simulink model "estimator"  (R2024b)
settings: Solver=VariableStepAuto  StartTime=0.0  StopTime=10.0  RelTol=1e-6
undefined symbols (not defined in the file): i, init, o
settings Model: Creator=jefft  LastModifiedBy=jefft
settings SFSimCC: SimCustomHeaderCode="#include \"estimator.h\""  SimTargetLang=C++
settings SFSimCC: SimUserSources=|
  | MathFunctions.cpp
  | MEKF.cpp
  | MEKFEstimatorModule.cpp
  | estimator.cpp
settings SFSimCC: SimUserIncludeDirs=|
  | ../lib/math
  | ../lib/estimator
  | ../lib/error
  | ../lib/flightmodule
settings RTWCC: GPUComputeCapability=3.5

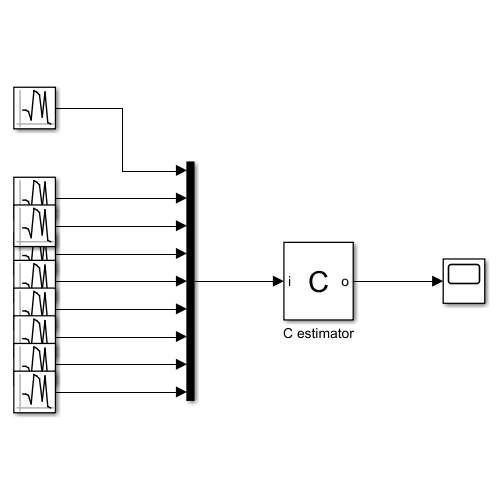
[thumbnail: Simulink's stored preview of the top-level diagram]
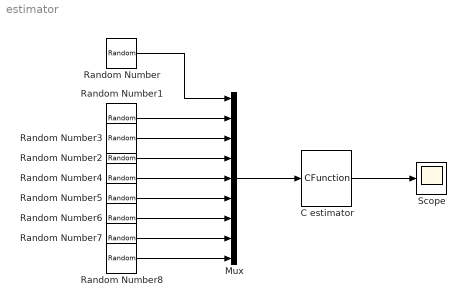
== system estimator ==
  C estimator : CFunction  OutputCode=run(i, o);  StartCode=init();  GenerateCodeAsIs=off  CodegenOutputCode=run(i, o);  CodegenStartCode=init();  CustomCodeSettingLocation=ModelConfigurationParameters
  Mux : Mux  Inputs=9
  Random Number : RandomNumber  Mean=1  Seed=1  SampleTime=0.1
  Random Number1 : RandomNumber  Mean=1  Seed=2  SampleTime=0.1
  Random Number2 : RandomNumber  Mean=1  Seed=5  SampleTime=0.1
  Random Number3 : RandomNumber  Mean=1  Seed=1  SampleTime=0.1
  Random Number4 : RandomNumber  Mean=1  SampleTime=0.1
  Random Number{5..8} (4 alike) : RandomNumber  Mean=1  Seed=6  SampleTime=0.1
  Scope : Scope
  wires:
  Mux/1 -> C estimator/1
  Random Number/1 -> Mux/1
  C estimator/1 -> Scope/1
  Random Number1/1 -> Mux/2
  Random Number2/1 -> Mux/4
  Random Number5/1 -> Mux/6
  Random Number4/1 -> Mux/5
  Random Number3/1 -> Mux/3
  Random Number6/1 -> Mux/7
  Random Number7/1 -> Mux/8
  Random Number8/1 -> Mux/9
